simulink model "DualUser_Haptic_TrainingSystem"  (R2022b)
settings: Solver=VariableStepAuto  StartTime=0.0  StopTime=5  RelTol=1e-3
libraries: cstblocks x1
settings Model: Creator=alire  LastModifiedBy=alire

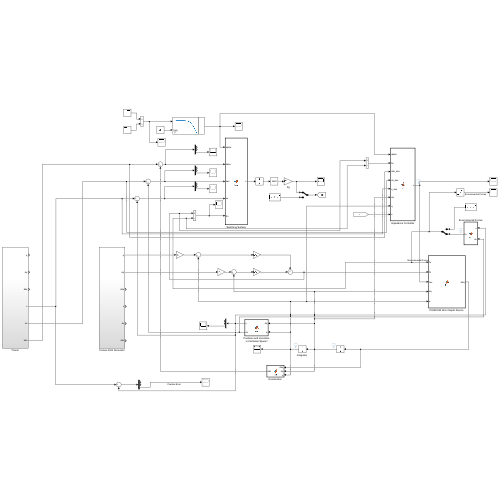
[thumbnail: Simulink's stored preview of the top-level diagram]
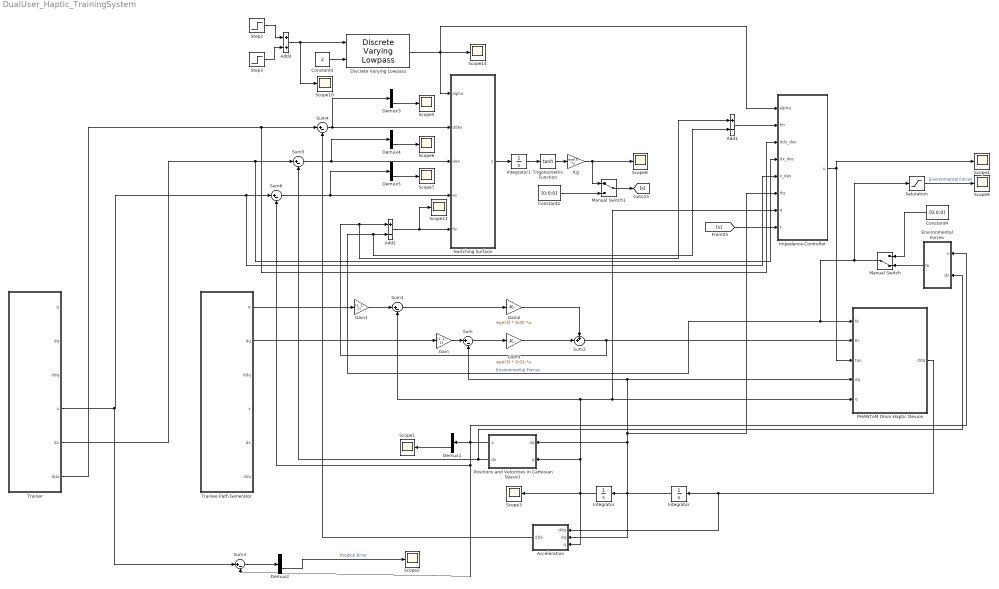
== system DualUser_Haptic_TrainingSystem ==
  "Acceleration " : MATLAB Function  TreatAsAtomicUnit=on
  Add1 : Sum  Inputs=+-
  Add2 : Sum  Inputs=+-
  Add3 : Sum
  Constant2 : Constant  Value=[0;0;0]
  Constant3 : Constant  Value=2
  Constant4 : Constant  Value=[0;0;0]
  Demux{1..5} (5 alike) : Demux  Outputs=3
  Discrete Varying Lowpass : cstblocks/Linear Parameter Varying/Discrete Varying Lowpass  N=1  w0=0  Ts=0.001
  Environmental Forces : MATLAB Function  TreatAsAtomicUnit=on
  Gain : Gain  Gain=[1; 1; 1]
  Gain1 : Gain  Gain=[1; 1; 1]
  Gain2 : Gain  Gain=eye(3) * 0.05  Multiplication=Matrix(K*u)
  Gain3 : Gain  Gain=eye(3) * 0.01  Multiplication=Matrix(K*u)
  Impedance Controller : MATLAB Function  TreatAsAtomicUnit=on
  Integrator : Integrator  InitialCondition=[0;0;0]
  "Integrator " : Integrator  InitialCondition="[-0.1746    0.7011    0.5365]'"
  Integrator1 : Integrator  InitialCondition=[0;0;0]
  Kg : Gain  Gain=eye(3)  Multiplication=Matrix(K*u)
  Manual Switch : ManualSwitch  CurrentSetting=0
  Manual Switch1 : ManualSwitch
  "PHANToM Omni Haptic Device " : MATLAB Function  TreatAsAtomicUnit=on
  Positions and Velocities in Cartesian Space1 : MATLAB Function  TreatAsAtomicUnit=on
  Saturation : Saturate  LowerLimit=0
  Scope{1..11,14} (12 alike) : Scope
  Step2 : Step  SampleTime=0
  Step3 : Step  Time=3  After=-1  SampleTime=0
  Sum{,1,3..6} (6 alike) : Sum  Inputs=|+-
  Sum2 : Sum  Inputs=++|
  Switching Surface : MATLAB Function  TreatAsAtomicUnit=on
  Trainee Path Generator : Subsystem
  Trainer : Subsystem
  Trigonometric Function : Trigonometry  Operator=tanh
  wires:
  Saturation/1 -> Scope9/1  "Environmental Forces"
  Constant4/1 -> Manual Switch/1
  Kg/1 -> Scope8/1, Manual Switch1/1
  Environmental Forces/1(fe) -> Manual Switch/2
  Positions and Velocities in Cartesian Space1/2(dx) -> Environmental Forces/2(dx), Sum5/2
  Trainee Path Generator/1(q) -> Gain1/1
  Manual Switch1/1 -> [s]
  "Integrator "/1 -> "Acceleration "/3(q), Scope3/1, Positions and Velocities in Cartesian Space1/2(q), Sum1/2, Impedance Controller/7(q), "PHANToM Omni Haptic Device "/5(q)
  Add3/1 -> Scope10/1, Discrete Varying Lowpass/1
  Sum6/1 -> Demux5/1, Switching Surface/4(ex)
  Constant2/1 -> Manual Switch1/2
  Sum1/1 -> Gain2/1
  Sum3/1 -> Demux2/1
  Add1/1 -> Impedance Controller/2(fm)
  Positions and Velocities in Cartesian Space1/1(x) -> Environmental Forces/1(x), Sum3/2, Sum6/2, Demux1/1
  Trainer/6(ddx) -> Impedance Controller/3(ddx_des), Sum4/1
  Step3/1 -> Add3/2
  Demux3/3 -> Scope5/1
  Sum5/1 -> Demux4/1, Switching Surface/3(dex)
  Gain/1 -> Sum/1
  Demux5/3 -> Scope7/1
  Step2/1 -> Add3/1
  [s] -> Impedance Controller/8(s)
  Demux4/3 -> Scope6/1
  Sum4/1 -> Switching Surface/2(ddex), Demux3/1
  Sum2/1 -> Add1/1, Add2/1, "PHANToM Omni Haptic Device "/2(fh)
  Gain3/1 -> Sum2/2
  Add2/1 -> Scope11/1, Switching Surface/5(fm)
  Trainer/5(dx) -> Impedance Controller/4(dx_des), Sum5/1
  Demux2/3 -> Scope2/1  "Position Error"
  Manual Switch/1 -> Saturation/1, Add1/2, Add2/2, "PHANToM Omni Haptic Device "/1(fe)  "Environmental Forces"
  Discrete Varying Lowpass/1 -> Switching Surface/1(alpha), Scope14/1, Impedance Controller/1(alpha)
  Switching Surface/1(s) -> Integrator1/1
  Integrator1/1 -> Trigonometric Function/1
  "Acceleration "/1(ddx) -> Sum4/2
  Impedance Controller/1(u) -> "PHANToM Omni Haptic Device "/3(tau), Scope4/1
  Integrator/1 -> "Acceleration "/2(dq), "Integrator "/1, Positions and Velocities in Cartesian Space1/1(dq), Sum/2, "PHANToM Omni Haptic Device "/4(dq), Impedance Controller/6(dq)
  Trainee Path Generator/2(dq) -> Gain/1
  Demux1/3 -> Scope1/1
  Sum/1 -> Gain3/1
  Trigonometric Function/1 -> Kg/1
  Gain1/1 -> Sum1/1
  Constant3/1 -> Discrete Varying Lowpass/2
  Trainer/4(x) -> Sum3/1, Impedance Controller/5(x_des), Sum6/1
  "PHANToM Omni Haptic Device "/1(ddq) -> "Acceleration "/1(ddq), Integrator/1
  Gain2/1 -> Sum2/1

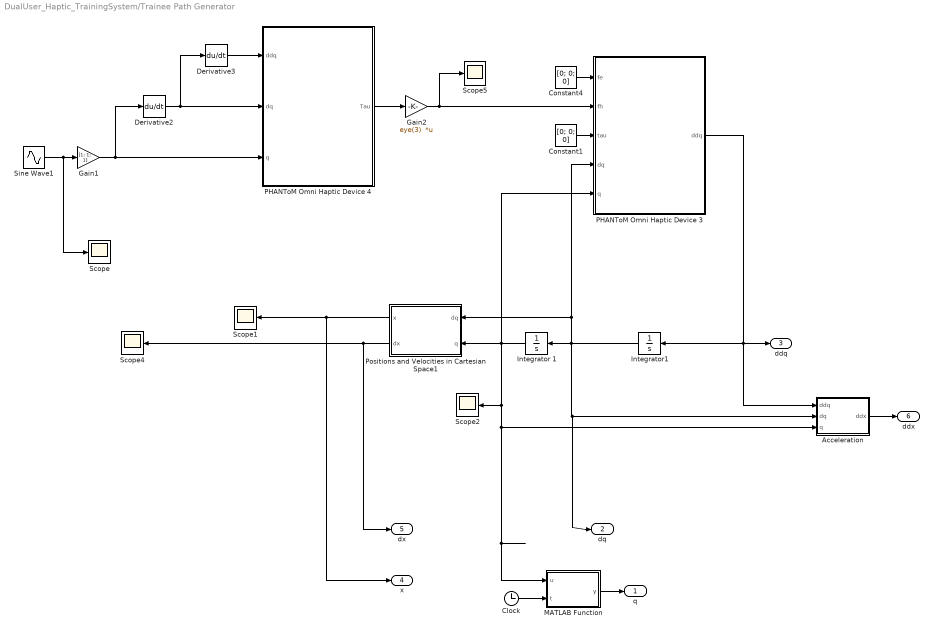
== system DualUser_Haptic_TrainingSystem/Trainee Path Generator ==
  "Acceleration " : MATLAB Function  TreatAsAtomicUnit=on
  Clock : Clock
  Constant1 : Constant  Value=[0; 0; 0]
  Constant4 : Constant  Value=[0; 0; 0]
  Derivative2 : Derivative
  Derivative3 : Derivative
  Gain1 : Gain  Gain=[1; 1; 1]
  Gain2 : Gain  Gain=eye(3)  Multiplication=Matrix(K*u)
  Integrator 1 : Integrator  InitialCondition="[-0.1746    0.7011    0.5365]'"
  Integrator1 : Integrator  InitialCondition=[0;0;0]
  MATLAB Function : MATLAB Function  TreatAsAtomicUnit=on
  PHANToM Omni Haptic Device 3 : MATLAB Function  TreatAsAtomicUnit=on
  PHANToM Omni Haptic Device 4 : MATLAB Function  TreatAsAtomicUnit=on
  Positions and Velocities in Cartesian Space1 : MATLAB Function  TreatAsAtomicUnit=on
  Scope{,1..2,4..5} (5 alike) : Scope
  Sine Wave1 : Sin  Amplitude=0.01  Frequency=0.5  SampleTime=0
  q : Outport  VectorParamsAs1DForOutWhenUnconnected=off
  dq : Outport  Port=2  VectorParamsAs1DForOutWhenUnconnected=off
  ddq : Outport  Port=3  VectorParamsAs1DForOutWhenUnconnected=off
  x : Outport  Port=4  VectorParamsAs1DForOutWhenUnconnected=off
  dx : Outport  Port=5  VectorParamsAs1DForOutWhenUnconnected=off
  ddx : Outport  Port=6  VectorParamsAs1DForOutWhenUnconnected=off
  wires:
  Positions and Velocities in Cartesian Space1/2(dx) -> dx/1, Scope4/1
  Positions and Velocities in Cartesian Space1/1(x) -> x/1, Scope1/1
  "Acceleration "/1(ddx) -> ddx/1
  Derivative3/1 -> PHANToM Omni Haptic Device 4/1(ddq)
  Integrator1/1 -> dq/1, "Acceleration "/2(dq), Integrator 1/1, PHANToM Omni Haptic Device 3/4(dq), Positions and Velocities in Cartesian Space1/1(dq)
  Gain2/1 -> Scope5/1, PHANToM Omni Haptic Device 3/2(fh)
  Constant4/1 -> PHANToM Omni Haptic Device 3/1(fe)
  Constant1/1 -> PHANToM Omni Haptic Device 3/3(tau)
  PHANToM Omni Haptic Device 4/1(Tau) -> Gain2/1
  Sine Wave1/1 -> Scope/1, Gain1/1
  PHANToM Omni Haptic Device 3/1(ddq) -> "Acceleration "/1(ddq), Integrator1/1, ddq/1
  Gain1/1 -> PHANToM Omni Haptic Device 4/3(q), Derivative2/1
  Derivative2/1 -> Derivative3/1, PHANToM Omni Haptic Device 4/2(dq)
  Clock/1 -> MATLAB Function/2(t)
  Integrator 1/1 -> PHANToM Omni Haptic Device 3/5(q), MATLAB Function/1(u), "Acceleration "/3(q), Scope2/1, Positions and Velocities in Cartesian Space1/2(q)
  MATLAB Function/1(y) -> q/1

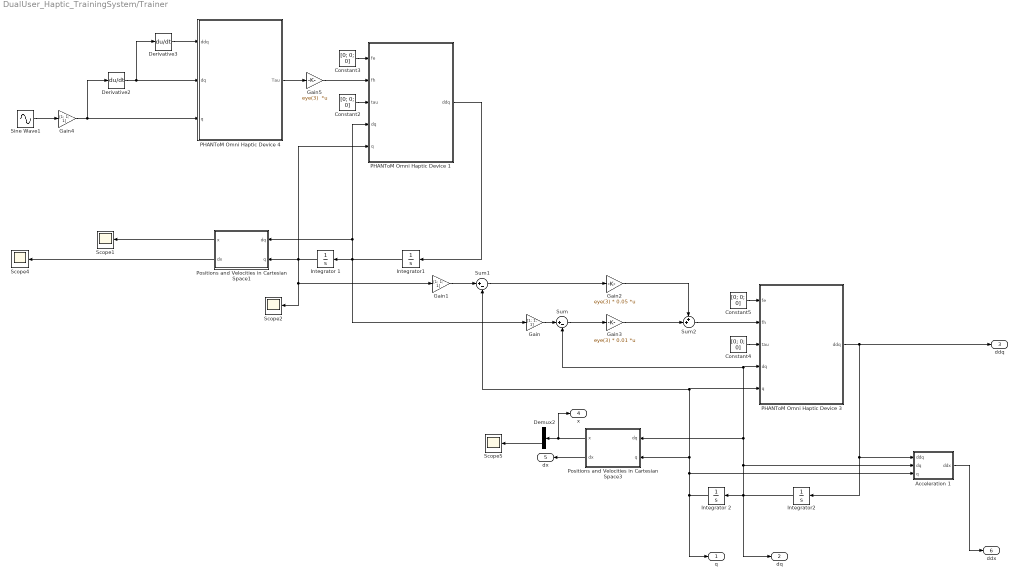
== system DualUser_Haptic_TrainingSystem/Trainer ==
  Acceleration 1 : MATLAB Function  TreatAsAtomicUnit=on
  Constant{2..5} (4 alike) : Constant  Value=[0; 0; 0]
  Demux2 : Demux  Outputs=3
  Derivative2 : Derivative
  Derivative3 : Derivative
  Gain : Gain  Gain=[1; 1; 1]
  Gain1 : Gain  Gain=[1; 1; 1]
  Gain2 : Gain  Gain=eye(3) * 0.05  Multiplication=Matrix(K*u)
  Gain3 : Gain  Gain=eye(3) * 0.01  Multiplication=Matrix(K*u)
  Gain4 : Gain  Gain=[1; 1; 1]
  Gain5 : Gain  Gain=eye(3)  Multiplication=Matrix(K*u)
  Integrator 1 : Integrator  InitialCondition="[-0.1746    0.7011    0.5365]'"
  Integrator 2 : Integrator  InitialCondition="[-0.1746    0.7011    0.5365]'"
  Integrator1 : Integrator  InitialCondition=[0;0;0]
  Integrator2 : Integrator  InitialCondition=[0;0;0]
  PHANToM Omni Haptic Device 1 : MATLAB Function  TreatAsAtomicUnit=on
  PHANToM Omni Haptic Device 3 : MATLAB Function  TreatAsAtomicUnit=on
  PHANToM Omni Haptic Device 4 : MATLAB Function  TreatAsAtomicUnit=on
  Positions and Velocities in Cartesian Space1 : MATLAB Function  TreatAsAtomicUnit=on
  Positions and Velocities in Cartesian Space3 : MATLAB Function  TreatAsAtomicUnit=on
  Scope{1..2,4..5} (4 alike) : Scope
  Sine Wave1 : Sin  Amplitude=0.01  Frequency=0.5  SampleTime=0
  Sum : Sum  Inputs=|+-
  Sum1 : Sum  Inputs=|+-
  Sum2 : Sum  Inputs=++|
  q : Outport  VectorParamsAs1DForOutWhenUnconnected=off
  dq : Outport  Port=2  VectorParamsAs1DForOutWhenUnconnected=off
  ddq : Outport  Port=3  VectorParamsAs1DForOutWhenUnconnected=off
  x : Outport  Port=4  VectorParamsAs1DForOutWhenUnconnected=off
  dx : Outport  Port=5  VectorParamsAs1DForOutWhenUnconnected=off
  ddx : Outport  Port=6  VectorParamsAs1DForOutWhenUnconnected=off
  wires:
  PHANToM Omni Haptic Device 1/1(ddq) -> Integrator1/1
  Positions and Velocities in Cartesian Space1/2(dx) -> Scope4/1
  Positions and Velocities in Cartesian Space1/1(x) -> Scope1/1
  Constant2/1 -> PHANToM Omni Haptic Device 1/3(tau)
  Constant3/1 -> PHANToM Omni Haptic Device 1/1(fe)
  Gain5/1 -> PHANToM Omni Haptic Device 1/2(fh)
  Integrator1/1 -> Gain/1, Integrator 1/1, Positions and Velocities in Cartesian Space1/1(dq), PHANToM Omni Haptic Device 1/4(dq)
  Demux2/3 -> Scope5/1
  Gain3/1 -> Sum2/2
  Integrator 1/1 -> Gain1/1, Scope2/1, Positions and Velocities in Cartesian Space1/2(q), PHANToM Omni Haptic Device 1/5(q)
  Gain2/1 -> Sum2/1
  Sum1/1 -> Gain2/1
  Positions and Velocities in Cartesian Space3/1(x) -> x/1, Demux2/1
  Sum/1 -> Gain3/1
  Constant5/1 -> PHANToM Omni Haptic Device 3/1(fe)
  Gain/1 -> Sum/1
  Constant4/1 -> PHANToM Omni Haptic Device 3/3(tau)
  Gain1/1 -> Sum1/1
  Sum2/1 -> PHANToM Omni Haptic Device 3/2(fh)
  Positions and Velocities in Cartesian Space3/2(dx) -> dx/1
  Integrator 2/1 -> q/1, Acceleration 1/3(q), Positions and Velocities in Cartesian Space3/2(q), Sum1/2, PHANToM Omni Haptic Device 3/5(q)
  Acceleration 1/1(ddx) -> ddx/1
  PHANToM Omni Haptic Device 3/1(ddq) -> ddq/1, Acceleration 1/1(ddq), Integrator2/1
  Integrator2/1 -> dq/1, Integrator 2/1, Acceleration 1/2(dq), Positions and Velocities in Cartesian Space3/1(dq), Sum/2, PHANToM Omni Haptic Device 3/4(dq)
  Sine Wave1/1 -> Gain4/1
  Derivative3/1 -> PHANToM Omni Haptic Device 4/1(ddq)
  Derivative2/1 -> Derivative3/1, PHANToM Omni Haptic Device 4/2(dq)
  PHANToM Omni Haptic Device 4/1(Tau) -> Gain5/1
  Gain4/1 -> Derivative2/1, PHANToM Omni Haptic Device 4/3(q)

== matlab function DualUser_Haptic_TrainingSystem/Trainee Path Generator/MATLAB Function ==
  data: u input; y output; t input
function y = fcn(u, t)
    if t > 1 && t < 1.01
        u(3) = u(3) + 10;
    end
    y = u;
end

== matlab function DualUser_Haptic_TrainingSystem/PHANToM Omni Haptic Device  ==
  data: fe input; fh input; ddq output; tau input; dq input; q input
function ddq = fcn(fe, fh, tau, dq, q)
q1 = q(1);
q2 = q(2);
q3 = q(3);
dq1 = dq(1);
dq2 = dq(2);
dq3 = dq(3);

k1 = 1.798e-3;
k2 = 0.864e-3;
k3 = 0.486e-3;
k4 = 2.766e-3;
k5 = 0.308e-3;
k6 = 2.526e-3;
k7 = 0.652e-3;
k8 = 164.158e-3;
k9 = 94.50e-3;
k10 = 117.294e-3;

l1 = 133.35e-3;
l2 = 133.35e-3;

j11 = -cos(q1)*(l2*sin(q3)+l1*cos(q2));
j12 = l2*sin(q1)*sin(q2);
j13 = -l2*sin(q1)*cos(q3);
j21 = 0;
j22 = l1*cos(q2);
j23 = l2*sin(q3);
j31 = -l2*sin(q1)*sin(q3)-l1*sin(q1)*cos(q2);
j32 = -l1*sin(q2)*cos(q1);
j33 = l2*cos(q1)*cos(q3);

J = [j11 j12 j13;j21 j22 j23;j31 j32 j33];

m11 = k1+k2*cos(2*q2)+k3*cos(2*q3)+k4*cos(q2)*sin(q3);
m12 = k5*sin(q2);
m13 = 0;
m21 = k5*sin(q2);
m22 = k6;
m23 = -0.5*k4*sin(q2-q3);
m31 = 0;
m32 = -0.5*k4*sin(q2-q3);
m33 = k7;

v11 = -k2*dq2*sin(2*q2)-k3*dq3*sin(2*q3)-0.5*k4*dq2*sin(q2)*sin(q3)+0.5*k4*dq3*cos(q2)*cos(q3);
v12 = -k2*dq1*sin(2*q2)+k5*dq2*cos(q2)-0.5*k4*dq1*sin(q2)*sin(q3);
v13 = -k3*dq1*sin(2*q3)+0.5*k4*dq1*cos(q2)*cos(q3);
v21 = k2*dq1*sin(2*q2)+0.5*k4*dq1*sin(q2)*sin(q3);
v22 = 0;
v23 = 0.5*k4*dq3*cos(q2-q3);
v31 = k3*dq1*sin(2*q3)+0.5*k4*dq1*cos(q2)*cos(q3);
v32 = -0.5*k4*dq2*cos(q2-q3);
v33 = 0;

n1 = 0;
n2 = k8*cos(q2)+k10*(q2-0.5*pi);
n3 = k9*sin(q3);

M = [m11 m12 m13;m21 m22 m23;m31 m32 m33];
V = [v11 v12 v13;v21 v22 v23; v31 v32 v33];
N = [n1;n2;n3];

ddq = M \ (-V*dq-N+J'*tau+(fh-fe));
end

== matlab function DualUser_Haptic_TrainingSystem/Trainer/Positions and Velocities in Cartesian Space1 ==
  data: dq input; q input; x output; dx output
function [x, dx] = fcn(dq, q)
q1 = q(1);
q2 = q(2);
q3 = q(3);
dq1 = dq(1);
dq2 = dq(2);
dq3 = dq(3);

l1 = 133.35e-3;
l2 = 133.35e-3;
l3 = 23.35e-3;
l4 = 168.35e-3;

j11 = -cos(q1)*(l2*sin(q3)+l1*cos(q2));
j12 = l2*sin(q1)*sin(q2);
j13 = -l2*sin(q1)*cos(q3);
j21 = 0;
j22 = l1*cos(q2);
j23 = l2*sin(q3);
j31 = -l2*sin(q1)*sin(q3)-l1*sin(q1)*cos(q2);
j32 = -l1*sin(q2)*cos(q1);
j33 = l2*cos(q1)*cos(q3);

dj11 = sin(q1)*dq1*(l2*sin(q3)+l1*cos(q2))-(l2*cos(q3)*dq3-l1*sin(q2)*dq2)*cos(q1);
dj12 = l2*cos(q1)*dq1*sin(q2)+cos(q2)*dq2*l2*sin(q1);
dj13 = -l2*cos(q1)*dq1*cos(q3)+sin(q3)*dq3*l2*sin(q1);
dj21 = 0;
dj22 = -l1*sin(q2)*dq2;
dj23 = l2*cos(q3)*dq3;
dj31 = -l2*cos(q1)*dq1*sin(q3)-cos(q3)*dq3*l2*sin(q1)-l1*cos(q1)*dq1*cos(q2)+sin(q2)*dq2*l1*sin(q1);
dj32 = -l1*cos(q2)*dq2*cos(q1)+sin(q1)*dq1*l1*sin(q2);
dj33 = -l2*sin(q1)*dq1*cos(q3)-sin(q3)*dq3*l2*cos(q1);

J = [j11 j12 j13;j21 j22 j23;j31 j32 j33];
dJ = [dj11 dj12 dj13;dj21 dj22 dj23;dj31 dj32 dj33];

x1 = -sin(q1)*(l2*sin(q3)+l1*cos(q2));
x2 = -l2*cos(q3)+l1*sin(q2)+l3;
x3 = l2*cos(q1)*sin(q3)+l1*cos(q1)*cos(q2)-l4;

x = [x1;x2;x3];
dx = J*dq;
% ddx = dJ*dq+J*ddq;
end

== matlab function DualUser_Haptic_TrainingSystem/Impedance Controller ==
  data: alpha input; fm input; ddx_des input; u output; dx_des input; x_des input; dq input; q input; s input
function u = fcn(alpha, fm, ddx_des, dx_des, x_des, dq, q, s)
q1 = q(1);
q2 = q(2);
q3 = q(3);
dq1 = dq(1);
dq2 = dq(2);
dq3 = dq(3);

k1 = 1.798e-3;
k2 = 0.864e-3;
k3 = 0.486e-3;
k4 = 2.766e-3;
k5 = 0.308e-3;
k6 = 2.526e-3;
k7 = 0.652e-3;
k8 = 164.158e-3;
k9 = 94.50e-3;
k10 = 117.294e-3;

l1 = 133.35e-3;
l2 = 133.35e-3;
l3 = 23.35e-3;
l4 = 168.35e-3;

j11 = -cos(q1)*(l2*sin(q3)+l1*cos(q2));
j12 = l2*sin(q1)*sin(q2);
j13 = -l2*sin(q1)*cos(q3);
j21 = 0;
j22 = l1*cos(q2);
j23 = l2*sin(q3);
j31 = -l2*sin(q1)*sin(q3)-l1*sin(q1)*cos(q2);
j32 = -l1*sin(q2)*cos(q1);
j33 = l2*cos(q1)*cos(q3);

dj11 = sin(q1)*dq1*(l2*sin(q3)+l1*cos(q2))-(l2*cos(q3)*dq3-l1*sin(q2)*dq2)*cos(q1);
dj12 = l2*cos(q1)*dq1*sin(q2)+cos(q2)*dq2*l2*sin(q1);
dj13 = -l2*cos(q1)*dq1*cos(q3)+sin(q3)*dq3*l2*sin(q1);
dj21 = 0;
dj22 = -l1*sin(q2)*dq2;
dj23 = l2*cos(q3)*dq3;
dj31 = -l2*cos(q1)*dq1*sin(q3)-cos(q3)*dq3*l2*sin(q1)-l1*cos(q1)*dq1*cos(q2)+sin(q2)*dq2*l1*sin(q1);
dj32 = -l1*cos(q2)*dq2*cos(q1)+sin(q1)*dq1*l1*sin(q2);
dj33 = -l2*sin(q1)*dq1*cos(q3)-sin(q3)*dq3*l2*cos(q1);

J = [j11 j12 j13;j21 j22 j23;j31 j32 j33];
dJ = [dj11 dj12 dj13;dj21 dj22 dj23;dj31 dj32 dj33];

x1 = -sin(q1)*(l2*sin(q3)+l1*cos(q2));
x2 = -l2*cos(q3)+l1*sin(q2)+l3;
x3 = l2*cos(q1)*sin(q3)+l1*cos(q1)*cos(q2)-l4;

x = [x1;x2;x3];
dx = J*dq;

m11 = k1+k2*cos(2*q2)+k3*cos(2*q3)+k4*cos(q2)*sin(q3);
m12 = k5*sin(q2);
m13 = 0;
m21 = k5*sin(q2);
m22 = k6;
m23 = -0.5*k4*sin(q2-q3);
m31 = 0;
m32 = -0.5*k4*sin(q2-q3);
m33 = k7;

v11 = -k2*dq2*sin(2*q2)-k3*dq3*sin(2*q3)-0.5*k4*dq2*sin(q2)*sin(q3)+0.5*k4*dq3*cos(q2)*cos(q3);
v12 = -k2*dq1*sin(2*q2)+k5*dq2*cos(q2)-0.5*k4*dq1*sin(q2)*sin(q3);
v13 = -k3*dq1*sin(2*q3)+0.5*k4*dq1*cos(q2)*cos(q3);
v21 = k2*dq1*sin(2*q2)+0.5*k4*dq1*sin(q2)*sin(q3);
v22 = 0;
v23 = 0.5*k4*dq3*cos(q2-q3);
v31 = k3*dq1*sin(2*q3)+0.5*k4*dq1*cos(q2)*cos(q3);
v32 = -0.5*k4*dq2*cos(q2-q3);
v33 = 0;

n1 = 0;
n2 = k8*cos(q2)+k10*(q2-0.5*pi);
n3 = k9*sin(q3);

M = [m11 m12 m13;m21 m22 m23;m31 m32 m33];
V = [v11 v12 v13;v21 v22 v23; v31 v32 v33];
N = [n1;n2;n3];

D = inv(J')*M*inv(J);
C = inv(J')*(V-M*inv(J)*dJ)*inv(J);
G = inv(J')*N;

Md = alpha*0.001*eye(3)+(1-alpha)*0.1*eye(3);
Bd = alpha*40*eye(3)+(1-alpha)*4*eye(3);
Kd = alpha*1000*eye(3)+(1-alpha)*100*eye(3);

e = x_des-x;
de = dx_des-dx;

u = D*(inv(Md)*(Md*ddx_des+Kd*e+Bd*de-fm)+s)+(C*dx+G-fm);
end

== matlab function DualUser_Haptic_TrainingSystem/Trainee Path Generator/PHANToM Omni Haptic Device 3 ==
  data: fe input; fh input; ddq output; tau input; dq input; q input
function ddq = fcn(fe, fh, tau, dq, q)
q1 = q(1);
q2 = q(2);
q3 = q(3);
dq1 = dq(1);
dq2 = dq(2);
dq3 = dq(3);

k1 = 1.798e-3;
k2 = 0.864e-3;
k3 = 0.486e-3;
k4 = 2.766e-3;
k5 = 0.308e-3;
k6 = 2.526e-3;
k7 = 0.652e-3;
k8 = 164.158e-3;
k9 = 94.50e-3;
k10 = 117.294e-3;

l1 = 133.35e-3;
l2 = 133.35e-3;

j11 = -cos(q1)*(l2*sin(q3)+l1*cos(q2));
j12 = l2*sin(q1)*sin(q2);
j13 = -l2*sin(q1)*cos(q3);
j21 = 0;
j22 = l1*cos(q2);
j23 = l2*sin(q3);
j31 = -l2*sin(q1)*sin(q3)-l1*sin(q1)*cos(q2);
j32 = -l1*sin(q2)*cos(q1);
j33 = l2*cos(q1)*cos(q3);

J = [j11 j12 j13;j21 j22 j23;j31 j32 j33];

m11 = k1+k2*cos(2*q2)+k3*cos(2*q3)+k4*cos(q2)*sin(q3);
m12 = k5*sin(q2);
m13 = 0;
m21 = k5*sin(q2);
m22 = k6;
m23 = -0.5*k4*sin(q2-q3);
m31 = 0;
m32 = -0.5*k4*sin(q2-q3);
m33 = k7;

v11 = -k2*dq2*sin(2*q2)-k3*dq3*sin(2*q3)-0.5*k4*dq2*sin(q2)*sin(q3)+0.5*k4*dq3*cos(q2)*cos(q3);
v12 = -k2*dq1*sin(2*q2)+k5*dq2*cos(q2)-0.5*k4*dq1*sin(q2)*sin(q3);
v13 = -k3*dq1*sin(2*q3)+0.5*k4*dq1*cos(q2)*cos(q3);
v21 = k2*dq1*sin(2*q2)+0.5*k4*dq1*sin(q2)*sin(q3);
v22 = 0;
v23 = 0.5*k4*dq3*cos(q2-q3);
v31 = k3*dq1*sin(2*q3)+0.5*k4*dq1*cos(q2)*cos(q3);
v32 = -0.5*k4*dq2*cos(q2-q3);
v33 = 0;

n1 = 0;
n2 = k8*cos(q2)+k10*(q2-0.5*pi);
n3 = k9*sin(q3);

M = [m11 m12 m13;m21 m22 m23;m31 m32 m33];
V = [v11 v12 v13;v21 v22 v23; v31 v32 v33];
N = [n1;n2;n3];

ddq = M \ (-V*dq-N+J'*tau+(fh-fe));
end

== matlab function DualUser_Haptic_TrainingSystem/Trainee Path Generator/PHANToM Omni Haptic Device 4 ==
  data: ddq input; Tau output; dq input; q input
function Tau = fcn(ddq, dq, q)
q1 = q(1);
q2 = q(2);
q3 = q(3);
dq1 = dq(1);
dq2 = dq(2);
dq3 = dq(3);

k1 = 1.798e-3;
k2 = 0.864e-3;
k3 = 0.486e-3;
k4 = 2.766e-3;
k5 = 0.308e-3;
k6 = 2.526e-3;
k7 = 0.652e-3;
k8 = 164.158e-3;
k9 = 94.50e-3;
k10 = 117.294e-3;

l1 = 133.35e-3;
l2 = 133.35e-3;

j11 = -cos(q1)*(l2*sin(q3)+l1*cos(q2));
j12 = l2*sin(q1)*sin(q2);
j13 = -l2*sin(q1)*cos(q3);
j21 = 0;
j22 = l1*cos(q2);
j23 = l2*sin(q3);
j31 = -l2*sin(q1)*sin(q3)-l1*sin(q1)*cos(q2);
j32 = -l1*sin(q2)*cos(q1);
j33 = l2*cos(q1)*cos(q3);

J = [j11 j12 j13;j21 j22 j23;j31 j32 j33];

m11 = k1+k2*cos(2*q2)+k3*cos(2*q3)+k4*cos(q2)*sin(q3);
m12 = k5*sin(q2);
m13 = 0;
m21 = k5*sin(q2);
m22 = k6;
m23 = -0.5*k4*sin(q2-q3);
m31 = 0;
m32 = -0.5*k4*sin(q2-q3);
m33 = k7;

v11 = -k2*dq2*sin(2*q2)-k3*dq3*sin(2*q3)-0.5*k4*dq2*sin(q2)*sin(q3)+0.5*k4*dq3*cos(q2)*cos(q3);
v12 = -k2*dq1*sin(2*q2)+k5*dq2*cos(q2)-0.5*k4*dq1*sin(q2)*sin(q3);
v13 = -k3*dq1*sin(2*q3)+0.5*k4*dq1*cos(q2)*cos(q3);
v21 = k2*dq1*sin(2*q2)+0.5*k4*dq1*sin(q2)*sin(q3);
v22 = 0;
v23 = 0.5*k4*dq3*cos(q2-q3);
v31 = k3*dq1*sin(2*q3)+0.5*k4*dq1*cos(q2)*cos(q3);
v32 = -0.5*k4*dq2*cos(q2-q3);
v33 = 0;

n1 = 0;
n2 = k8*cos(q2)+k10*(q2-0.5*pi);
n3 = k9*sin(q3);

M = [m11 m12 m13;m21 m22 m23;m31 m32 m33];
V = [v11 v12 v13;v21 v22 v23; v31 v32 v33];
N = [n1;n2;n3];

Tau = M * ddq + V * dq + N;
end

== matlab function DualUser_Haptic_TrainingSystem/Trainer/Acceleration 1 ==
  data: ddq input; ddx output; dq input; q input
function ddx = fcn(ddq, dq, q)
q1 = q(1);
q2 = q(2);
q3 = q(3);
dq1 = dq(1);
dq2 = dq(2);
dq3 = dq(3);

l1 = 133.35e-3;
l2 = 133.35e-3;
l3 = 23.35e-3;
l4 = 168.35e-3;

j11 = -cos(q1)*(l2*sin(q3)+l1*cos(q2));
j12 = l2*sin(q1)*sin(q2);
j13 = -l2*sin(q1)*cos(q3);
j21 = 0;
j22 = l1*cos(q2);
j23 = l2*sin(q3);
j31 = -l2*sin(q1)*sin(q3)-l1*sin(q1)*cos(q2);
j32 = -l1*sin(q2)*cos(q1);
j33 = l2*cos(q1)*cos(q3);

dj11 = sin(q1)*dq1*(l2*sin(q3)+l1*cos(q2))-(l2*cos(q3)*dq3-l1*sin(q2)*dq2)*cos(q1);
dj12 = l2*cos(q1)*dq1*sin(q2)+cos(q2)*dq2*l2*sin(q1);
dj13 = -l2*cos(q1)*dq1*cos(q3)+sin(q3)*dq3*l2*sin(q1);
dj21 = 0;
dj22 = -l1*sin(q2)*dq2;
dj23 = l2*cos(q3)*dq3;
dj31 = -l2*cos(q1)*dq1*sin(q3)-cos(q3)*dq3*l2*sin(q1)-l1*cos(q1)*dq1*cos(q2)+sin(q2)*dq2*l1*sin(q1);
dj32 = -l1*cos(q2)*dq2*cos(q1)+sin(q1)*dq1*l1*sin(q2);
dj33 = -l2*sin(q1)*dq1*cos(q3)-sin(q3)*dq3*l2*cos(q1);

J = [j11 j12 j13;j21 j22 j23;j31 j32 j33];
dJ = [dj11 dj12 dj13;dj21 dj22 dj23;dj31 dj32 dj33];

x1 = -sin(q1)*(l2*sin(q3)+l1*cos(q2));
x2 = -l2*cos(q3)+l1*sin(q2)+l3;
x3 = l2*cos(q1)*sin(q3)+l1*cos(q1)*cos(q2)-l4;

x = [x1;x2;x3];
dx = J*dq;
ddx = J*ddq+dJ*dq;
end

== matlab function DualUser_Haptic_TrainingSystem/Switching Surface ==
  data: alpha input; ddex input; s output; dex input; ex input; fm input
function s = fcn(alpha, ddex, dex, ex, fm)
Md = alpha * 0.001 * eye(3) + (1 - alpha) * 0.1 * eye(3);
Bd = alpha * 40 * eye(3) + (1 - alpha) * 4 * eye(3);
Kd = alpha * 1000 * eye(3) + (1 - alpha) * 100 * eye(3);

s = ddex + Md \ (Bd * dex + Kd * ex - fm);
end

== matlab function DualUser_Haptic_TrainingSystem/Trainer/PHANToM Omni Haptic Device 4 ==
  data: ddq input; Tau output; dq input; q input
function Tau = fcn(ddq, dq, q)
q1 = q(1);
q2 = q(2);
q3 = q(3);
dq1 = dq(1);
dq2 = dq(2);
dq3 = dq(3);

k1 = 1.798e-3;
k2 = 0.864e-3;
k3 = 0.486e-3;
k4 = 2.766e-3;
k5 = 0.308e-3;
k6 = 2.526e-3;
k7 = 0.652e-3;
k8 = 164.158e-3;
k9 = 94.50e-3;
k10 = 117.294e-3;

l1 = 133.35e-3;
l2 = 133.35e-3;

j11 = -cos(q1)*(l2*sin(q3)+l1*cos(q2));
j12 = l2*sin(q1)*sin(q2);
j13 = -l2*sin(q1)*cos(q3);
j21 = 0;
j22 = l1*cos(q2);
j23 = l2*sin(q3);
j31 = -l2*sin(q1)*sin(q3)-l1*sin(q1)*cos(q2);
j32 = -l1*sin(q2)*cos(q1);
j33 = l2*cos(q1)*cos(q3);

J = [j11 j12 j13;j21 j22 j23;j31 j32 j33];

m11 = k1+k2*cos(2*q2)+k3*cos(2*q3)+k4*cos(q2)*sin(q3);
m12 = k5*sin(q2);
m13 = 0;
m21 = k5*sin(q2);
m22 = k6;
m23 = -0.5*k4*sin(q2-q3);
m31 = 0;
m32 = -0.5*k4*sin(q2-q3);
m33 = k7;

v11 = -k2*dq2*sin(2*q2)-k3*dq3*sin(2*q3)-0.5*k4*dq2*sin(q2)*sin(q3)+0.5*k4*dq3*cos(q2)*cos(q3);
v12 = -k2*dq1*sin(2*q2)+k5*dq2*cos(q2)-0.5*k4*dq1*sin(q2)*sin(q3);
v13 = -k3*dq1*sin(2*q3)+0.5*k4*dq1*cos(q2)*cos(q3);
v21 = k2*dq1*sin(2*q2)+0.5*k4*dq1*sin(q2)*sin(q3);
v22 = 0;
v23 = 0.5*k4*dq3*cos(q2-q3);
v31 = k3*dq1*sin(2*q3)+0.5*k4*dq1*cos(q2)*cos(q3);
v32 = -0.5*k4*dq2*cos(q2-q3);
v33 = 0;

n1 = 0;
n2 = k8*cos(q2)+k10*(q2-0.5*pi);
n3 = k9*sin(q3);

M = [m11 m12 m13;m21 m22 m23;m31 m32 m33];
V = [v11 v12 v13;v21 v22 v23; v31 v32 v33];
N = [n1;n2;n3];

Tau = M * ddq + V * dq + N;
end

== matlab function DualUser_Haptic_TrainingSystem/Acceleration  ==
  data: ddq input; ddx output; dq input; q input
function ddx = fcn(ddq, dq, q)
q1 = q(1);
q2 = q(2);
q3 = q(3);
dq1 = dq(1);
dq2 = dq(2);
dq3 = dq(3);

l1 = 133.35e-3;
l2 = 133.35e-3;
l3 = 23.35e-3;
l4 = 168.35e-3;

j11 = -cos(q1)*(l2*sin(q3)+l1*cos(q2));
j12 = l2*sin(q1)*sin(q2);
j13 = -l2*sin(q1)*cos(q3);
j21 = 0;
j22 = l1*cos(q2);
j23 = l2*sin(q3);
j31 = -l2*sin(q1)*sin(q3)-l1*sin(q1)*cos(q2);
j32 = -l1*sin(q2)*cos(q1);
j33 = l2*cos(q1)*cos(q3);

dj11 = sin(q1)*dq1*(l2*sin(q3)+l1*cos(q2))-(l2*cos(q3)*dq3-l1*sin(q2)*dq2)*cos(q1);
dj12 = l2*cos(q1)*dq1*sin(q2)+cos(q2)*dq2*l2*sin(q1);
dj13 = -l2*cos(q1)*dq1*cos(q3)+sin(q3)*dq3*l2*sin(q1);
dj21 = 0;
dj22 = -l1*sin(q2)*dq2;
dj23 = l2*cos(q3)*dq3;
dj31 = -l2*cos(q1)*dq1*sin(q3)-cos(q3)*dq3*l2*sin(q1)-l1*cos(q1)*dq1*cos(q2)+sin(q2)*dq2*l1*sin(q1);
dj32 = -l1*cos(q2)*dq2*cos(q1)+sin(q1)*dq1*l1*sin(q2);
dj33 = -l2*sin(q1)*dq1*cos(q3)-sin(q3)*dq3*l2*cos(q1);

J = [j11 j12 j13;j21 j22 j23;j31 j32 j33];
dJ = [dj11 dj12 dj13;dj21 dj22 dj23;dj31 dj32 dj33];

x1 = -sin(q1)*(l2*sin(q3)+l1*cos(q2));
x2 = -l2*cos(q3)+l1*sin(q2)+l3;
x3 = l2*cos(q1)*sin(q3)+l1*cos(q1)*cos(q2)-l4;

x = [x1;x2;x3];
dx = J*dq;
ddx = J*ddq+dJ*dq;
end

== matlab function DualUser_Haptic_TrainingSystem/Trainer/PHANToM Omni Haptic Device 1 ==
  data: fe input; fh input; ddq output; tau input; dq input; q input
function ddq = fcn(fe, fh, tau, dq, q)
q1 = q(1);
q2 = q(2);
q3 = q(3);
dq1 = dq(1);
dq2 = dq(2);
dq3 = dq(3);

k1 = 1.798e-3;
k2 = 0.864e-3;
k3 = 0.486e-3;
k4 = 2.766e-3;
k5 = 0.308e-3;
k6 = 2.526e-3;
k7 = 0.652e-3;
k8 = 164.158e-3;
k9 = 94.50e-3;
k10 = 117.294e-3;

l1 = 133.35e-3;
l2 = 133.35e-3;

j11 = -cos(q1)*(l2*sin(q3)+l1*cos(q2));
j12 = l2*sin(q1)*sin(q2);
j13 = -l2*sin(q1)*cos(q3);
j21 = 0;
j22 = l1*cos(q2);
j23 = l2*sin(q3);
j31 = -l2*sin(q1)*sin(q3)-l1*sin(q1)*cos(q2);
j32 = -l1*sin(q2)*cos(q1);
j33 = l2*cos(q1)*cos(q3);

J = [j11 j12 j13;j21 j22 j23;j31 j32 j33];

m11 = k1+k2*cos(2*q2)+k3*cos(2*q3)+k4*cos(q2)*sin(q3);
m12 = k5*sin(q2);
m13 = 0;
m21 = k5*sin(q2);
m22 = k6;
m23 = -0.5*k4*sin(q2-q3);
m31 = 0;
m32 = -0.5*k4*sin(q2-q3);
m33 = k7;

v11 = -k2*dq2*sin(2*q2)-k3*dq3*sin(2*q3)-0.5*k4*dq2*sin(q2)*sin(q3)+0.5*k4*dq3*cos(q2)*cos(q3);
v12 = -k2*dq1*sin(2*q2)+k5*dq2*cos(q2)-0.5*k4*dq1*sin(q2)*sin(q3);
v13 = -k3*dq1*sin(2*q3)+0.5*k4*dq1*cos(q2)*cos(q3);
v21 = k2*dq1*sin(2*q2)+0.5*k4*dq1*sin(q2)*sin(q3);
v22 = 0;
v23 = 0.5*k4*dq3*cos(q2-q3);
v31 = k3*dq1*sin(2*q3)+0.5*k4*dq1*cos(q2)*cos(q3);
v32 = -0.5*k4*dq2*cos(q2-q3);
v33 = 0;

n1 = 0;
n2 = k8*cos(q2)+k10*(q2-0.5*pi);
n3 = k9*sin(q3);

M = [m11 m12 m13;m21 m22 m23;m31 m32 m33];
V = [v11 v12 v13;v21 v22 v23; v31 v32 v33];
N = [n1;n2;n3];

ddq = M \ (-V*dq-N+J'*tau+(fh-fe));
end

== matlab function DualUser_Haptic_TrainingSystem/Positions and Velocities in Cartesian Space1 ==
  data: dq input; q input; x output; dx output
function [x, dx] = fcn(dq, q)
q1 = q(1);
q2 = q(2);
q3 = q(3);
dq1 = dq(1);
dq2 = dq(2);
dq3 = dq(3);

l1 = 133.35e-3;
l2 = 133.35e-3;
l3 = 23.35e-3;
l4 = 168.35e-3;

j11 = -cos(q1)*(l2*sin(q3)+l1*cos(q2));
j12 = l2*sin(q1)*sin(q2);
j13 = -l2*sin(q1)*cos(q3);
j21 = 0;
j22 = l1*cos(q2);
j23 = l2*sin(q3);
j31 = -l2*sin(q1)*sin(q3)-l1*sin(q1)*cos(q2);
j32 = -l1*sin(q2)*cos(q1);
j33 = l2*cos(q1)*cos(q3);

dj11 = sin(q1)*dq1*(l2*sin(q3)+l1*cos(q2))-(l2*cos(q3)*dq3-l1*sin(q2)*dq2)*cos(q1);
dj12 = l2*cos(q1)*dq1*sin(q2)+cos(q2)*dq2*l2*sin(q1);
dj13 = -l2*cos(q1)*dq1*cos(q3)+sin(q3)*dq3*l2*sin(q1);
dj21 = 0;
dj22 = -l1*sin(q2)*dq2;
dj23 = l2*cos(q3)*dq3;
dj31 = -l2*cos(q1)*dq1*sin(q3)-cos(q3)*dq3*l2*sin(q1)-l1*cos(q1)*dq1*cos(q2)+sin(q2)*dq2*l1*sin(q1);
dj32 = -l1*cos(q2)*dq2*cos(q1)+sin(q1)*dq1*l1*sin(q2);
dj33 = -l2*sin(q1)*dq1*cos(q3)-sin(q3)*dq3*l2*cos(q1);

J = [j11 j12 j13;j21 j22 j23;j31 j32 j33];
dJ = [dj11 dj12 dj13;dj21 dj22 dj23;dj31 dj32 dj33];

x1 = -sin(q1)*(l2*sin(q3)+l1*cos(q2));
x2 = -l2*cos(q3)+l1*sin(q2)+l3;
x3 = l2*cos(q1)*sin(q3)+l1*cos(q1)*cos(q2)-l4;

x = [x1;x2;x3];
dx = J*dq;
% ddx = dJ*dq+J*ddq;
end

== matlab function DualUser_Haptic_TrainingSystem/Trainee Path Generator/Acceleration  ==
  data: ddq input; ddx output; dq input; q input
function ddx = fcn(ddq, dq, q)
q1 = q(1);
q2 = q(2);
q3 = q(3);
dq1 = dq(1);
dq2 = dq(2);
dq3 = dq(3);

l1 = 133.35e-3;
l2 = 133.35e-3;
l3 = 23.35e-3;
l4 = 168.35e-3;

j11 = -cos(q1)*(l2*sin(q3)+l1*cos(q2));
j12 = l2*sin(q1)*sin(q2);
j13 = -l2*sin(q1)*cos(q3);
j21 = 0;
j22 = l1*cos(q2);
j23 = l2*sin(q3);
j31 = -l2*sin(q1)*sin(q3)-l1*sin(q1)*cos(q2);
j32 = -l1*sin(q2)*cos(q1);
j33 = l2*cos(q1)*cos(q3);

dj11 = sin(q1)*dq1*(l2*sin(q3)+l1*cos(q2))-(l2*cos(q3)*dq3-l1*sin(q2)*dq2)*cos(q1);
dj12 = l2*cos(q1)*dq1*sin(q2)+cos(q2)*dq2*l2*sin(q1);
dj13 = -l2*cos(q1)*dq1*cos(q3)+sin(q3)*dq3*l2*sin(q1);
dj21 = 0;
dj22 = -l1*sin(q2)*dq2;
dj23 = l2*cos(q3)*dq3;
dj31 = -l2*cos(q1)*dq1*sin(q3)-cos(q3)*dq3*l2*sin(q1)-l1*cos(q1)*dq1*cos(q2)+sin(q2)*dq2*l1*sin(q1);
dj32 = -l1*cos(q2)*dq2*cos(q1)+sin(q1)*dq1*l1*sin(q2);
dj33 = -l2*sin(q1)*dq1*cos(q3)-sin(q3)*dq3*l2*cos(q1);

J = [j11 j12 j13;j21 j22 j23;j31 j32 j33];
dJ = [dj11 dj12 dj13;dj21 dj22 dj23;dj31 dj32 dj33];

x1 = -sin(q1)*(l2*sin(q3)+l1*cos(q2));
x2 = -l2*cos(q3)+l1*sin(q2)+l3;
x3 = l2*cos(q1)*sin(q3)+l1*cos(q1)*cos(q2)-l4;

x = [x1;x2;x3];
dx = J*dq;
ddx = J*ddq+dJ*dq;
end

== matlab function DualUser_Haptic_TrainingSystem/Trainer/PHANToM Omni Haptic Device 3 ==
  data: fe input; fh input; ddq output; tau input; dq input; q input
function ddq = fcn(fe, fh, tau, dq, q)
q1 = q(1);
q2 = q(2);
q3 = q(3);
dq1 = dq(1);
dq2 = dq(2);
dq3 = dq(3);

k1 = 1.798e-3;
k2 = 0.864e-3;
k3 = 0.486e-3;
k4 = 2.766e-3;
k5 = 0.308e-3;
k6 = 2.526e-3;
k7 = 0.652e-3;
k8 = 164.158e-3;
k9 = 94.50e-3;
k10 = 117.294e-3;

l1 = 133.35e-3;
l2 = 133.35e-3;

j11 = -cos(q1)*(l2*sin(q3)+l1*cos(q2));
j12 = l2*sin(q1)*sin(q2);
j13 = -l2*sin(q1)*cos(q3);
j21 = 0;
j22 = l1*cos(q2);
j23 = l2*sin(q3);
j31 = -l2*sin(q1)*sin(q3)-l1*sin(q1)*cos(q2);
j32 = -l1*sin(q2)*cos(q1);
j33 = l2*cos(q1)*cos(q3);

J = [j11 j12 j13;j21 j22 j23;j31 j32 j33];

m11 = k1+k2*cos(2*q2)+k3*cos(2*q3)+k4*cos(q2)*sin(q3);
m12 = k5*sin(q2);
m13 = 0;
m21 = k5*sin(q2);
m22 = k6;
m23 = -0.5*k4*sin(q2-q3);
m31 = 0;
m32 = -0.5*k4*sin(q2-q3);
m33 = k7;

v11 = -k2*dq2*sin(2*q2)-k3*dq3*sin(2*q3)-0.5*k4*dq2*sin(q2)*sin(q3)+0.5*k4*dq3*cos(q2)*cos(q3);
v12 = -k2*dq1*sin(2*q2)+k5*dq2*cos(q2)-0.5*k4*dq1*sin(q2)*sin(q3);
v13 = -k3*dq1*sin(2*q3)+0.5*k4*dq1*cos(q2)*cos(q3);
v21 = k2*dq1*sin(2*q2)+0.5*k4*dq1*sin(q2)*sin(q3);
v22 = 0;
v23 = 0.5*k4*dq3*cos(q2-q3);
v31 = k3*dq1*sin(2*q3)+0.5*k4*dq1*cos(q2)*cos(q3);
v32 = -0.5*k4*dq2*cos(q2-q3);
v33 = 0;

n1 = 0;
n2 = k8*cos(q2)+k10*(q2-0.5*pi);
n3 = k9*sin(q3);

M = [m11 m12 m13;m21 m22 m23;m31 m32 m33];
V = [v11 v12 v13;v21 v22 v23; v31 v32 v33];
N = [n1;n2;n3];

ddq = M \ (-V*dq-N+J'*tau+(fh-fe));
end

== matlab function DualUser_Haptic_TrainingSystem/Trainer/Positions and Velocities in Cartesian Space3 ==
  data: dq input; q input; x output; dx output
function [x, dx] = fcn(dq, q)
q1 = q(1);
q2 = q(2);
q3 = q(3);
dq1 = dq(1);
dq2 = dq(2);
dq3 = dq(3);

l1 = 133.35e-3;
l2 = 133.35e-3;
l3 = 23.35e-3;
l4 = 168.35e-3;

j11 = -cos(q1)*(l2*sin(q3)+l1*cos(q2));
j12 = l2*sin(q1)*sin(q2);
j13 = -l2*sin(q1)*cos(q3);
j21 = 0;
j22 = l1*cos(q2);
j23 = l2*sin(q3);
j31 = -l2*sin(q1)*sin(q3)-l1*sin(q1)*cos(q2);
j32 = -l1*sin(q2)*cos(q1);
j33 = l2*cos(q1)*cos(q3);

dj11 = sin(q1)*dq1*(l2*sin(q3)+l1*cos(q2))-(l2*cos(q3)*dq3-l1*sin(q2)*dq2)*cos(q1);
dj12 = l2*cos(q1)*dq1*sin(q2)+cos(q2)*dq2*l2*sin(q1);
dj13 = -l2*cos(q1)*dq1*cos(q3)+sin(q3)*dq3*l2*sin(q1);
dj21 = 0;
dj22 = -l1*sin(q2)*dq2;
dj23 = l2*cos(q3)*dq3;
dj31 = -l2*cos(q1)*dq1*sin(q3)-cos(q3)*dq3*l2*sin(q1)-l1*cos(q1)*dq1*cos(q2)+sin(q2)*dq2*l1*sin(q1);
dj32 = -l1*cos(q2)*dq2*cos(q1)+sin(q1)*dq1*l1*sin(q2);
dj33 = -l2*sin(q1)*dq1*cos(q3)-sin(q3)*dq3*l2*cos(q1);

J = [j11 j12 j13;j21 j22 j23;j31 j32 j33];
dJ = [dj11 dj12 dj13;dj21 dj22 dj23;dj31 dj32 dj33];

x1 = -sin(q1)*(l2*sin(q3)+l1*cos(q2));
x2 = -l2*cos(q3)+l1*sin(q2)+l3;
x3 = l2*cos(q1)*sin(q3)+l1*cos(q1)*cos(q2)-l4;

x = [x1;x2;x3];
dx = J*dq;
% ddx = dJ*dq+J*ddq;
end

== matlab function DualUser_Haptic_TrainingSystem/Trainee Path Generator/Positions and Velocities in Cartesian Space1 ==
  data: dq input; q input; x output; dx output
function [x, dx] = fcn(dq, q)
q1 = q(1);
q2 = q(2);
q3 = q(3);
dq1 = dq(1);
dq2 = dq(2);
dq3 = dq(3);

l1 = 133.35e-3;
l2 = 133.35e-3;
l3 = 23.35e-3;
l4 = 168.35e-3;

j11 = -cos(q1)*(l2*sin(q3)+l1*cos(q2));
j12 = l2*sin(q1)*sin(q2);
j13 = -l2*sin(q1)*cos(q3);
j21 = 0;
j22 = l1*cos(q2);
j23 = l2*sin(q3);
j31 = -l2*sin(q1)*sin(q3)-l1*sin(q1)*cos(q2);
j32 = -l1*sin(q2)*cos(q1);
j33 = l2*cos(q1)*cos(q3);

dj11 = sin(q1)*dq1*(l2*sin(q3)+l1*cos(q2))-(l2*cos(q3)*dq3-l1*sin(q2)*dq2)*cos(q1);
dj12 = l2*cos(q1)*dq1*sin(q2)+cos(q2)*dq2*l2*sin(q1);
dj13 = -l2*cos(q1)*dq1*cos(q3)+sin(q3)*dq3*l2*sin(q1);
dj21 = 0;
dj22 = -l1*sin(q2)*dq2;
dj23 = l2*cos(q3)*dq3;
dj31 = -l2*cos(q1)*dq1*sin(q3)-cos(q3)*dq3*l2*sin(q1)-l1*cos(q1)*dq1*cos(q2)+sin(q2)*dq2*l1*sin(q1);
dj32 = -l1*cos(q2)*dq2*cos(q1)+sin(q1)*dq1*l1*sin(q2);
dj33 = -l2*sin(q1)*dq1*cos(q3)-sin(q3)*dq3*l2*cos(q1);

J = [j11 j12 j13;j21 j22 j23;j31 j32 j33];
dJ = [dj11 dj12 dj13;dj21 dj22 dj23;dj31 dj32 dj33];

x1 = -sin(q1)*(l2*sin(q3)+l1*cos(q2));
x2 = -l2*cos(q3)+l1*sin(q2)+l3;
x3 = l2*cos(q1)*sin(q3)+l1*cos(q1)*cos(q2)-l4;

x = [x1;x2;x3];
dx = J*dq;
% ddx = dJ*dq+J*ddq;
end

== matlab function DualUser_Haptic_TrainingSystem/Environmental Forces ==
  data: x input; fe output; dx input
function fe = fcn(x, dx)
if (x(3)>0)
    fe = [0;0;1*x(3)+0.2*dx(3)];
else
    fe = [0;0;0];
end    
end
